simulink library "legs"  (R2020b)
settings: Solver=VariableStepAuto  StartTime=0.0  StopTime=10.0  RelTol=1e-3
values from neighbouring files (symbols this model uses):
  N = size(waypoints, 1)    [interpolate_leg_waypoints.m]
undefined symbols (not defined in the file or in its folder): beta, X, Y, Z
libraries: sm_lib x42, $bdroot x21, nesl_utility x9
(part 1 of 2)
settings Model: Creator=zach  LastModifiedBy=zach

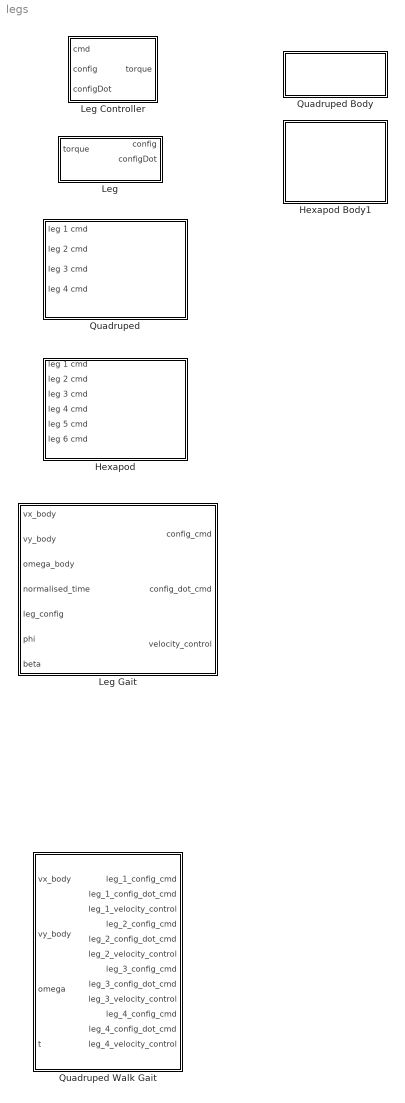
== system legs ==
  Hexapod : Subsystem  AncestorBlock=legs/Quadruped
  Hexapod Body1 : Subsystem  AncestorBlock=legs/Quadruped Body  mask{radius=0.5, height=0.1, leg_radius=0.02, mass=0}
      mask prompts: leg_radius "Leg Radius"
  Leg : Subsystem  mask{length_1=0.1, length_2=0.3, length_3=0.3, radius=0.04, mass_1=0.1, mass_2=0.3, mass_3=0.3}
      mask prompts: length_1 "Length 1"; length_2 "Length 2"; length_3 "Length 3"; mass_1 "Mass 1"; mass_2 "Mass 2"; mass_3 "Mass 3"
  Leg Controller : Subsystem  mask{kp=[10; 10; 10], ki=[1; 1; 1], kd=[0.1; 0.1; 0.1]}
  Leg Gait : Subsystem  mask{distance=0.3, rotation_z=0, contact_start_config=[0; pi/4; pi/4]}
      mask prompts: rotation_z "Rotation Z"; contact_start_config "Leg config at start of contact phase"
  Quadruped : Subsystem
  Quadruped Body : Subsystem  mask{length=0.4, width=0.3, height=0.1, leg_radius=0.04, mass=0}
      mask prompts: leg_radius "Leg Radius"
  Quadruped Walk Gait : Subsystem  mask{T=1}
      mask prompts: T "Period"

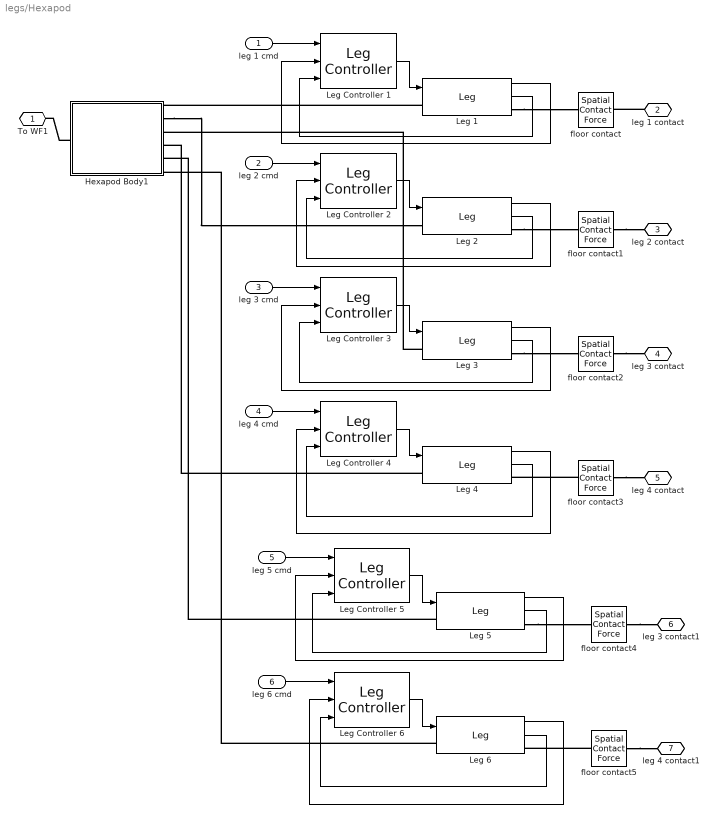
== system legs/Hexapod ==
  leg 1 cmd : Inport
  leg 2 cmd : Inport  Port=2
  leg 3 cmd : Inport  Port=3
  leg 4 cmd : Inport  Port=4
  leg 5 cmd : Inport  Port=5
  leg 6 cmd : Inport  Port=6
  Hexapod Body1 : Subsystem  AncestorBlock=legs/Quadruped Body  mask{radius=0.5, height=0.1, leg_radius=0.02, mass=0}
      mask prompts: leg_radius "Leg Radius"
  Leg {1..6} (6 alike) : $bdroot/Leg  length_1=0.1  length_2=0.3  length_3=0.3  radius=0.02  mass_1=0.1  mass_2=0.3  mass_3=0.3
  Leg Controller {1..6} (6 alike) : $bdroot/Leg Controller  kp=[20; 20; 20]  ki=[5; 5; 5]  kd=[1; 1; 1]
  floor contact{,1..5} (6 alike) : sm_lib/Forces and Torques/Spatial Contact Force  CoefficientOfDynamicFriction=0.3  CoefficientOfStaticFriction=1  NormalDamping=1e3  NormalDampingUnits=N/(m/s)  NormalStiffness=1e6  NormalStiffnessUnits=N/m  FrictionalCriticalVelocity=1e-3  FrictionalCriticalVelocityUnits=m/s  ZeroCrossDetectContactStartAndEnd=off  SenseFrictionalForceMagnitude=off  SenseNormalForceMagnitude=off  SenseSeparationDistance=off  NormalTransitionRegionWidth=1e-4  NormalTransitionRegionWidthUnits=m  FrictionType=SmoothStickSlip
  To WF1 : PMIOPort  Side=Left
  leg 1 contact : PMIOPort  Port=2  Side=Right
  leg 2 contact : PMIOPort  Port=3  Side=Right
  leg 3 contact : PMIOPort  Port=4  Side=Right
  leg 4 contact : PMIOPort  Port=5  Side=Right
  leg 3 contact1 : PMIOPort  Port=6  Side=Right
  leg 4 contact1 : PMIOPort  Port=7  Side=Right
  wires:
  Leg 2/2 -> Leg Controller 2/3
  Leg 2/1 -> Leg Controller 2/2
  Leg 1/1 -> Leg Controller 1/2
  leg 2 cmd/1 -> Leg Controller 2/1
  Leg 3/2 -> Leg Controller 3/3
  leg 4 cmd/1 -> Leg Controller 4/1
  leg 1 cmd/1 -> Leg Controller 1/1
  leg 3 cmd/1 -> Leg Controller 3/1
  Leg 4/1 -> Leg Controller 4/2
  Leg Controller 4/1 -> Leg 4/1
  Leg 4/2 -> Leg Controller 4/3
  Leg 3/1 -> Leg Controller 3/2
  Leg Controller 1/1 -> Leg 1/1
  Leg 1/2 -> Leg Controller 1/3
  Leg Controller 3/1 -> Leg 3/1
  Leg Controller 2/1 -> Leg 2/1
  Leg Controller 5/1 -> Leg 5/1
  Leg 6/1 -> Leg Controller 6/2
  leg 5 cmd/1 -> Leg Controller 5/1
  Leg Controller 6/1 -> Leg 6/1
  Leg 6/2 -> Leg Controller 6/3
  Leg 5/2 -> Leg Controller 5/3
  leg 6 cmd/1 -> Leg Controller 6/1
  Leg 5/1 -> Leg Controller 5/2
  connections:
  floor contact1/RConn1 -- leg 2 contact/RConn1
  floor contact3/RConn1 -- leg 4 contact/RConn1
  floor contact2/RConn1 -- leg 3 contact/RConn1
  leg 1 contact/RConn1 -- floor contact/RConn1
  Leg 1/RConn1 -- floor contact/LConn1
  Leg 3/LConn1 -- Hexapod Body1/RConn3
  Hexapod Body1/RConn2 -- Leg 2/LConn1
  Leg 1/LConn1 -- Hexapod Body1/RConn1
  Leg 4/LConn1 -- Hexapod Body1/RConn4
  Leg 2/RConn1 -- floor contact1/LConn1
  floor contact3/LConn1 -- Leg 4/RConn1
  Leg 3/RConn1 -- floor contact2/LConn1
  Hexapod Body1/LConn1 -- To WF1/RConn1
  floor contact4/RConn1 -- leg 3 contact1/RConn1
  floor contact5/RConn1 -- leg 4 contact1/RConn1
  Leg 6/LConn1 -- Hexapod Body1/RConn6
  Leg 5/RConn1 -- floor contact4/LConn1
  floor contact5/LConn1 -- Leg 6/RConn1
  Leg 5/LConn1 -- Hexapod Body1/RConn5

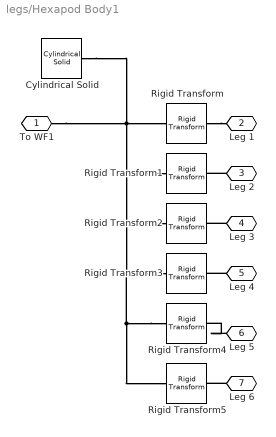
== system legs/Hexapod Body1 ==
  Cylindrical Solid : sm_lib/Body Elements/Cylindrical Solid  GraphicAmbientColor=[0.15 0.15 0.15 1.0]  BasedOnType=Density  CenterOfMass=[0 0 0]  CenterOfMassUnits=m  GraphicDiffuseColor=[0.5 0.5 0.5]  CylinderLength=height  CylinderLengthUnits=m  CylinderRadius=radius  CylinderRadiusUnits=m  Density=1000  DensityUnits=kg/m^3  DoExposeReferenceFrame=on  GraphicEmissiveColor=[0.0 0.0 0.0 1.0]  ExportEntireGeometry=off  SerializedFrames=<Frames/>  MarkerShape=Sphere  MarkerSize=10  GraphicType=FromGeometry  InertiaType=CalculateFromGeometry  Mass=1  MassUnits=kg  MomentsOfInertia=[1 1 1]  MomentsOfInertiaUnits=kg*m^2  GraphicOpacity=1.0  ProductsOfInertia=[0 0 0]  ProductsOfInertiaUnits=kg*m^2  GraphicShininess=75  GraphicSpecularColor=[0.5 0.5 0.5 1.0]  GraphicVisPropType=SimpleVisualProperties
  Rigid Transform : sm_lib/Frames and Transforms/Rigid Transform  TranslationMethod=Cylindrical  TranslationStandardOffset=0  TranslationLengthUnit=m  TranslationStandardAxis=+Z  TranslationCartesianOffset=[radius*cos(1/3*pi) radius*sin(1/3*pi) 0]  TranslationROffset=radius  TranslationROffsetUnits=m  TranslationZOffset=0  TranslationZOffsetUnits=m  TranslationThetaOffset=60  TranslationThetaOffsetUnits=deg  RotationMethod=StandardAxis  RotationAngleUnits=deg  RotationStandardAxis=+Z  RotationAngle=60  RotationArbitraryAxis=[0 0 1]  FollAlignAxisA=+X  BaseAlignAxisA=+Y  FollAlignAxisB=+Y  BaseAlignAxisB=+Z  RotationSequenceAxes=FollowerAxes  RotationSequence=XYX  RotationSequenceAngles=[0 0 0]  RotationSequenceAnglesUnits=deg  RotationMatrix=[1 0 0; 0 1 0; 0 0 1]
  Rigid Transform1 : sm_lib/Frames and Transforms/Rigid Transform  TranslationMethod=Cartesian  TranslationStandardOffset=0  TranslationLengthUnit=m  TranslationStandardAxis=+Z  TranslationCartesianOffset=[radius*cos(2/3*pi) radius*sin(2/3*pi) 0]  TranslationROffset=0  TranslationROffsetUnits=m  TranslationZOffset=0  TranslationZOffsetUnits=m  TranslationThetaOffset=0  TranslationThetaOffsetUnits=deg  RotationMethod=StandardAxis  RotationAngleUnits=rad  RotationStandardAxis=+Z  RotationAngle=2/3*pi  RotationArbitraryAxis=[0 0 1]  FollAlignAxisA=+X  BaseAlignAxisA=+Y  FollAlignAxisB=+Y  BaseAlignAxisB=+Z  RotationSequenceAxes=FollowerAxes  RotationSequence=XYX  RotationSequenceAngles=[0 0 0]  RotationSequenceAnglesUnits=deg  RotationMatrix=[1 0 0; 0 1 0; 0 0 1]
  Rigid Transform2 : sm_lib/Frames and Transforms/Rigid Transform  TranslationMethod=Cartesian  TranslationStandardOffset=0  TranslationLengthUnit=m  TranslationStandardAxis=+Z  TranslationCartesianOffset=[radius*cos(pi) radius*sin(pi) 0]  TranslationROffset=0  TranslationROffsetUnits=m  TranslationZOffset=0  TranslationZOffsetUnits=m  TranslationThetaOffset=0  TranslationThetaOffsetUnits=deg  RotationMethod=StandardAxis  RotationAngleUnits=rad  RotationStandardAxis=+Z  RotationAngle=pi  RotationArbitraryAxis=[0 0 1]  FollAlignAxisA=+X  BaseAlignAxisA=+Y  FollAlignAxisB=+Y  BaseAlignAxisB=+Z  RotationSequenceAxes=FollowerAxes  RotationSequence=XYX  RotationSequenceAngles=[0 0 0]  RotationSequenceAnglesUnits=deg  RotationMatrix=[1 0 0; 0 1 0; 0 0 1]
  Rigid Transform3 : sm_lib/Frames and Transforms/Rigid Transform  TranslationMethod=Cartesian  TranslationStandardOffset=0  TranslationLengthUnit=m  TranslationStandardAxis=+Z  TranslationCartesianOffset=[radius*cos(4/3*pi) radius*sin(4/3*pi) 0]  TranslationROffset=0  TranslationROffsetUnits=m  TranslationZOffset=0  TranslationZOffsetUnits=m  TranslationThetaOffset=0  TranslationThetaOffsetUnits=deg  RotationMethod=StandardAxis  RotationAngleUnits=rad  RotationStandardAxis=+Z  RotationAngle=4/3*pi  RotationArbitraryAxis=[0 0 1]  FollAlignAxisA=+X  BaseAlignAxisA=+Y  FollAlignAxisB=+Y  BaseAlignAxisB=+Z  RotationSequenceAxes=FollowerAxes  RotationSequence=XYX  RotationSequenceAngles=[0 0 0]  RotationSequenceAnglesUnits=deg  RotationMatrix=[1 0 0; 0 1 0; 0 0 1]
  Rigid Transform4 : sm_lib/Frames and Transforms/Rigid Transform  TranslationMethod=Cartesian  TranslationStandardOffset=0  TranslationLengthUnit=m  TranslationStandardAxis=+Z  TranslationCartesianOffset=[radius*cos(5/3*pi) radius*sin(5/3*pi) 0]  TranslationROffset=0  TranslationROffsetUnits=m  TranslationZOffset=0  TranslationZOffsetUnits=m  TranslationThetaOffset=0  TranslationThetaOffsetUnits=deg  RotationMethod=StandardAxis  RotationAngleUnits=rad  RotationStandardAxis=+Z  RotationAngle=5/3*pi  RotationArbitraryAxis=[0 0 1]  FollAlignAxisA=+X  BaseAlignAxisA=+Y  FollAlignAxisB=+Y  BaseAlignAxisB=+Z  RotationSequenceAxes=FollowerAxes  RotationSequence=XYX  RotationSequenceAngles=[0 0 0]  RotationSequenceAnglesUnits=deg  RotationMatrix=[1 0 0; 0 1 0; 0 0 1]
  Rigid Transform5 : sm_lib/Frames and Transforms/Rigid Transform  TranslationMethod=Cartesian  TranslationStandardOffset=0  TranslationLengthUnit=m  TranslationStandardAxis=+Z  TranslationCartesianOffset=[radius*cos(2*pi) radius*sin(2*pi) 0]  TranslationROffset=0  TranslationROffsetUnits=m  TranslationZOffset=0  TranslationZOffsetUnits=m  TranslationThetaOffset=0  TranslationThetaOffsetUnits=deg  RotationMethod=StandardAxis  RotationAngleUnits=rad  RotationStandardAxis=+Z  RotationAngle=2*pi  RotationArbitraryAxis=[0 0 1]  FollAlignAxisA=+X  BaseAlignAxisA=+Y  FollAlignAxisB=+Y  BaseAlignAxisB=+Z  RotationSequenceAxes=FollowerAxes  RotationSequence=XYX  RotationSequenceAngles=[0 0 0]  RotationSequenceAnglesUnits=deg  RotationMatrix=[1 0 0; 0 1 0; 0 0 1]
  To WF1 : PMIOPort  Side=Left
  Leg 1 : PMIOPort  Port=2  Side=Right
  Leg 2 : PMIOPort  Port=3  Side=Right
  Leg 3 : PMIOPort  Port=4  Side=Right
  Leg 4 : PMIOPort  Port=5  Side=Right
  Leg 5 : PMIOPort  Port=6  Side=Right
  Leg 6 : PMIOPort  Port=7  Side=Right
  connections:
  Rigid Transform/RConn1 -- Leg 1/RConn1
  Rigid Transform4/LConn1 -- Rigid Transform5/LConn1 -- To WF1/RConn1 -- Cylindrical Solid/RConn1 -- Rigid Transform/LConn1 -- Rigid Transform1/LConn1 -- Rigid Transform2/LConn1 -- Rigid Transform3/LConn1
  Leg 2/RConn1 -- Rigid Transform1/RConn1
  Leg 4/RConn1 -- Rigid Transform3/RConn1
  Leg 3/RConn1 -- Rigid Transform2/RConn1
  Leg 5/RConn1 -- Rigid Transform4/RConn1
  Leg 6/RConn1 -- Rigid Transform5/RConn1

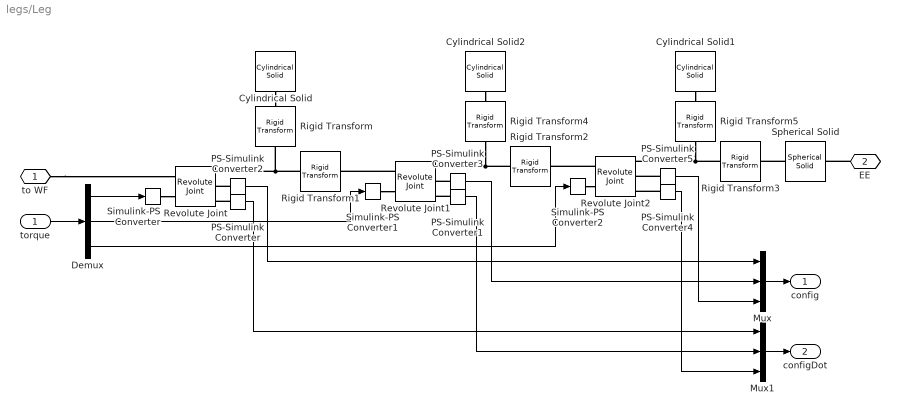
== system legs/Leg ==
  torque : Inport  PortDimensions=3
  Cylindrical Solid : sm_lib/Body Elements/Cylindrical Solid  GraphicAmbientColor=[0.15 0.15 0.15 1.0]  BasedOnType=Mass  CenterOfMass=[0 0 0]  CenterOfMassUnits=m  GraphicDiffuseColor=[0.2 0.2 0.2]  CylinderLength=length_1  CylinderLengthUnits=m  CylinderRadius=radius  CylinderRadiusUnits=m  Density=1000  DensityUnits=kg/m^3  DoExposeReferenceFrame=on  GraphicEmissiveColor=[0.0 0.0 0.0 1.0]  ExportEntireGeometry=off  SerializedFrames=<Frames/>  MarkerShape=Sphere  MarkerSize=10  GraphicType=FromGeometry  InertiaType=CalculateFromGeometry  Mass=mass_1  MassUnits=kg  MomentsOfInertia=[1 1 1]  MomentsOfInertiaUnits=kg*m^2  GraphicOpacity=1.0  ProductsOfInertia=[0 0 0]  ProductsOfInertiaUnits=kg*m^2  GraphicShininess=75  GraphicSpecularColor=[0.5 0.5 0.5 1.0]  GraphicVisPropType=SimpleVisualProperties
  Cylindrical Solid1 : sm_lib/Body Elements/Cylindrical Solid  GraphicAmbientColor=[0.15 0.15 0.15 1.0]  BasedOnType=Mass  CenterOfMass=[0 0 0]  CenterOfMassUnits=m  GraphicDiffuseColor=[0.2 0.2 0.2]  CylinderLength=length_3  CylinderLengthUnits=m  CylinderRadius=radius  CylinderRadiusUnits=m  Density=1000  DensityUnits=kg/m^3  DoExposeReferenceFrame=on  GraphicEmissiveColor=[0.0 0.0 0.0 1.0]  ExportEntireGeometry=off  SerializedFrames=<Frames/>  MarkerShape=Sphere  MarkerSize=10  GraphicType=FromGeometry  InertiaType=CalculateFromGeometry  Mass=mass_3  MassUnits=kg  MomentsOfInertia=[1 1 1]  MomentsOfInertiaUnits=kg*m^2  GraphicOpacity=1.0  ProductsOfInertia=[0 0 0]  ProductsOfInertiaUnits=kg*m^2  GraphicShininess=75  GraphicSpecularColor=[0.5 0.5 0.5 1.0]  GraphicVisPropType=SimpleVisualProperties
  Cylindrical Solid2 : sm_lib/Body Elements/Cylindrical Solid  GraphicAmbientColor=[0.15 0.15 0.15 1.0]  BasedOnType=Mass  CenterOfMass=[0 0 0]  CenterOfMassUnits=m  GraphicDiffuseColor=[0.2 0.2 0.2]  CylinderLength=length_2  CylinderLengthUnits=m  CylinderRadius=radius  CylinderRadiusUnits=m  Density=1000  DensityUnits=kg/m^3  DoExposeReferenceFrame=on  GraphicEmissiveColor=[0.0 0.0 0.0 1.0]  ExportEntireGeometry=off  SerializedFrames=<Frames/>  MarkerShape=Sphere  MarkerSize=10  GraphicType=FromGeometry  InertiaType=CalculateFromGeometry  Mass=mass_2  MassUnits=kg  MomentsOfInertia=[1 1 1]  MomentsOfInertiaUnits=kg*m^2  GraphicOpacity=1.0  ProductsOfInertia=[0 0 0]  ProductsOfInertiaUnits=kg*m^2  GraphicShininess=75  GraphicSpecularColor=[0.5 0.5 0.5 1.0]  GraphicVisPropType=SimpleVisualProperties
  Demux : Demux  Outputs=3
  Mux : Mux  Inputs=3
  Mux1 : Mux  Inputs=3
  PS-Simulink Converter{,1..5} (6 alike) : nesl_utility/PS-Simulink Converter  PhysicalDomain=network_engine_domain  SubClassName=ps_output  LeftPortType=input  RightPortType=output  PseudoPeriodic=off  Frequencies=[]  Unit=inherit  AffineConversion=off
  Revolute Joint : sm_lib/Joints/Revolute Joint  JointMode=Normal  SenseConstraintForce=off  SenseConstraintForceX=off  SenseConstraintForceY=off  SenseConstraintForceZ=off  SenseConstraintTorque=off  SenseConstraintTorqueX=off  SenseConstraintTorqueY=off  SenseConstraintTorqueZ=off  SenseTotalForce=off  SenseTotalForceX=off  SenseTotalForceY=off  SenseTotalForceZ=off  SenseTotalTorque=off  SenseTotalTorqueX=off  SenseTotalTorqueY=off  SenseTotalTorqueZ=off  CompositeWrenchDir=FollowerOnBase  CompositeWrenchFrame=BaseFrame  EquilibriumPosition=0  EquilibriumPositionUnits=deg  SpringStiffness=0  SpringStiffnessUnits=N*m/deg  DampingCoefficient=0  DampingCoefficientUnits=N*m/(deg/s)  TorqueActuationMode=InputTorque  MotionActuationMode=ComputedMotion  SensePosition=on  SenseVelocity=on  SenseAcceleration=off  SenseTorqueForce=off  SenseLowerLimitTorqueForce=off  SenseUpperLimitTorqueForce=off  LowerLimitSpecify=off  LowerLimitBound=-90  LowerLimitBoundUnits=deg  LowerLimitStiffness=1e4  LowerLimitStiffnessUnits=N*m/deg  LowerLimitDamping=10  LowerLimitDampingUnits=N*m/(deg/s)  LowerLimitTransitionRegionWidth=0.1  LowerLimitTransitionRegionWidthUnits=deg  UpperLimitSpecify=off  UpperLimitBound=90  UpperLimitBoundUnits=deg  UpperLimitStiffness=1e4  UpperLimitStiffnessUnits=N*m/deg  UpperLimitDamping=10  UpperLimitDampingUnits=N*m/(deg/s)  UpperLimitTransitionRegionWidth=0.1  UpperLimitTransitionRegionWidthUnits=deg  PositionTargetSpecify=on  PositionTargetPriority=High  PositionTargetValue=0  PositionTargetValueUnits=rad  VelocityTargetSpecify=on  VelocityTargetPriority=High  VelocityTargetValue=0  VelocityTargetValueUnits=deg/s
  Revolute Joint1 : sm_lib/Joints/Revolute Joint  JointMode=Normal  SenseConstraintForce=off  SenseConstraintForceX=off  SenseConstraintForceY=off  SenseConstraintForceZ=off  SenseConstraintTorque=off  SenseConstraintTorqueX=off  SenseConstraintTorqueY=off  SenseConstraintTorqueZ=off  SenseTotalForce=off  SenseTotalForceX=off  SenseTotalForceY=off  SenseTotalForceZ=off  SenseTotalTorque=off  SenseTotalTorqueX=off  SenseTotalTorqueY=off  SenseTotalTorqueZ=off  CompositeWrenchDir=FollowerOnBase  CompositeWrenchFrame=BaseFrame  EquilibriumPosition=0  EquilibriumPositionUnits=deg  SpringStiffness=0  SpringStiffnessUnits=N*m/deg  DampingCoefficient=0  DampingCoefficientUnits=N*m/(deg/s)  TorqueActuationMode=InputTorque  MotionActuationMode=ComputedMotion  SensePosition=on  SenseVelocity=on  SenseAcceleration=off  SenseTorqueForce=off  SenseLowerLimitTorqueForce=off  SenseUpperLimitTorqueForce=off  LowerLimitSpecify=off  LowerLimitBound=-90  LowerLimitBoundUnits=deg  LowerLimitStiffness=1e4  LowerLimitStiffnessUnits=N*m/deg  LowerLimitDamping=10  LowerLimitDampingUnits=N*m/(deg/s)  LowerLimitTransitionRegionWidth=0.1  LowerLimitTransitionRegionWidthUnits=deg  UpperLimitSpecify=off  UpperLimitBound=90  UpperLimitBoundUnits=deg  UpperLimitStiffness=1e4  UpperLimitStiffnessUnits=N*m/deg  UpperLimitDamping=10  UpperLimitDampingUnits=N*m/(deg/s)  UpperLimitTransitionRegionWidth=0.1  UpperLimitTransitionRegionWidthUnits=deg  PositionTargetSpecify=on  PositionTargetPriority=High  PositionTargetValue=0  PositionTargetValueUnits=rad  VelocityTargetSpecify=on  VelocityTargetPriority=High  VelocityTargetValue=0  VelocityTargetValueUnits=deg/s
  Revolute Joint2 : sm_lib/Joints/Revolute Joint  JointMode=Normal  SenseConstraintForce=off  SenseConstraintForceX=off  SenseConstraintForceY=off  SenseConstraintForceZ=off  SenseConstraintTorque=off  SenseConstraintTorqueX=off  SenseConstraintTorqueY=off  SenseConstraintTorqueZ=off  SenseTotalForce=off  SenseTotalForceX=off  SenseTotalForceY=off  SenseTotalForceZ=off  SenseTotalTorque=off  SenseTotalTorqueX=off  SenseTotalTorqueY=off  SenseTotalTorqueZ=off  CompositeWrenchDir=FollowerOnBase  CompositeWrenchFrame=BaseFrame  EquilibriumPosition=0  EquilibriumPositionUnits=deg  SpringStiffness=0  SpringStiffnessUnits=N*m/deg  DampingCoefficient=0  DampingCoefficientUnits=N*m/(deg/s)  TorqueActuationMode=InputTorque  MotionActuationMode=ComputedMotion  SensePosition=on  SenseVelocity=on  SenseAcceleration=off  SenseTorqueForce=off  SenseLowerLimitTorqueForce=off  SenseUpperLimitTorqueForce=off  LowerLimitSpecify=off  LowerLimitBound=-90  LowerLimitBoundUnits=deg  LowerLimitStiffness=1e4  LowerLimitStiffnessUnits=N*m/deg  LowerLimitDamping=10  LowerLimitDampingUnits=N*m/(deg/s)  LowerLimitTransitionRegionWidth=0.1  LowerLimitTransitionRegionWidthUnits=deg  UpperLimitSpecify=off  UpperLimitBound=90  UpperLimitBoundUnits=deg  UpperLimitStiffness=1e4  UpperLimitStiffnessUnits=N*m/deg  UpperLimitDamping=10  UpperLimitDampingUnits=N*m/(deg/s)  UpperLimitTransitionRegionWidth=0.1  UpperLimitTransitionRegionWidthUnits=deg  PositionTargetSpecify=on  PositionTargetPriority=High  PositionTargetValue=0  PositionTargetValueUnits=rad  VelocityTargetSpecify=on  VelocityTargetPriority=High  VelocityTargetValue=0  VelocityTargetValueUnits=deg/s
  Rigid Transform : sm_lib/Frames and Transforms/Rigid Transform  TranslationMethod=StandardAxis  TranslationStandardOffset=length_1/2  TranslationLengthUnit=m  TranslationStandardAxis=+Z  TranslationCartesianOffset=[0 0 0]  TranslationROffset=0  TranslationROffsetUnits=m  TranslationZOffset=0  TranslationZOffsetUnits=m  TranslationThetaOffset=0  TranslationThetaOffsetUnits=deg  RotationMethod=StandardAxis  RotationAngleUnits=deg  RotationStandardAxis=+Y  RotationAngle=90  RotationArbitraryAxis=[0 0 1]  FollAlignAxisA=+X  BaseAlignAxisA=+Y  FollAlignAxisB=+Y  BaseAlignAxisB=+Z  RotationSequenceAxes=FollowerAxes  RotationSequence=XYX  RotationSequenceAngles=[0 0 0]  RotationSequenceAnglesUnits=deg  RotationMatrix=[1 0 0; 0 1 0; 0 0 1]
  Rigid Transform1 : sm_lib/Frames and Transforms/Rigid Transform  TranslationMethod=StandardAxis  TranslationStandardOffset=length_1  TranslationLengthUnit=m  TranslationStandardAxis=+X  TranslationCartesianOffset=[0.1 0 0]  TranslationROffset=0  TranslationROffsetUnits=m  TranslationZOffset=0  TranslationZOffsetUnits=m  TranslationThetaOffset=0  TranslationThetaOffsetUnits=deg  RotationMethod=StandardAxis  RotationAngleUnits=deg  RotationStandardAxis=-X  RotationAngle=90  RotationArbitraryAxis=[0 0 1]  FollAlignAxisA=+X  BaseAlignAxisA=+Y  FollAlignAxisB=+Y  BaseAlignAxisB=+Z  RotationSequenceAxes=FollowerAxes  RotationSequence=XYX  RotationSequenceAngles=[0 0 0]  RotationSequenceAnglesUnits=deg  RotationMatrix=[1 0 0; 0 1 0; 0 0 1]
  Rigid Transform2 : sm_lib/Frames and Transforms/Rigid Transform  TranslationMethod=StandardAxis  TranslationStandardOffset=length_2  TranslationLengthUnit=m  TranslationStandardAxis=+X  TranslationCartesianOffset=[0 0 0]  TranslationROffset=0  TranslationROffsetUnits=m  TranslationZOffset=0  TranslationZOffsetUnits=m  TranslationThetaOffset=0  TranslationThetaOffsetUnits=deg  RotationMethod=None  RotationAngleUnits=deg  RotationStandardAxis=+X  RotationAngle=90  RotationArbitraryAxis=[0 0 1]  FollAlignAxisA=+X  BaseAlignAxisA=+Y  FollAlignAxisB=+Y  BaseAlignAxisB=+Z  RotationSequenceAxes=FollowerAxes  RotationSequence=XYX  RotationSequenceAngles=[0 0 0]  RotationSequenceAnglesUnits=deg  RotationMatrix=[1 0 0; 0 1 0; 0 0 1]
  Rigid Transform3 : sm_lib/Frames and Transforms/Rigid Transform  TranslationMethod=StandardAxis  TranslationStandardOffset=length_3  TranslationLengthUnit=m  TranslationStandardAxis=+X  TranslationCartesianOffset=[0 0 0]  TranslationROffset=0  TranslationROffsetUnits=m  TranslationZOffset=0  TranslationZOffsetUnits=m  TranslationThetaOffset=0  TranslationThetaOffsetUnits=deg  RotationMethod=None  RotationAngleUnits=deg  RotationStandardAxis=+X  RotationAngle=90  RotationArbitraryAxis=[0 0 1]  FollAlignAxisA=+X  BaseAlignAxisA=+Y  FollAlignAxisB=+Y  BaseAlignAxisB=+Z  RotationSequenceAxes=FollowerAxes  RotationSequence=XYX  RotationSequenceAngles=[0 0 0]  RotationSequenceAnglesUnits=deg  RotationMatrix=[1 0 0; 0 1 0; 0 0 1]
  Rigid Transform4 : sm_lib/Frames and Transforms/Rigid Transform  TranslationMethod=StandardAxis  TranslationStandardOffset=length_2/2  TranslationLengthUnit=m  TranslationStandardAxis=+Z  TranslationCartesianOffset=[0 0 0]  TranslationROffset=0  TranslationROffsetUnits=m  TranslationZOffset=0  TranslationZOffsetUnits=m  TranslationThetaOffset=0  TranslationThetaOffsetUnits=deg  RotationMethod=StandardAxis  RotationAngleUnits=deg  RotationStandardAxis=+Y  RotationAngle=90  RotationArbitraryAxis=[0 0 1]  FollAlignAxisA=+X  BaseAlignAxisA=+Y  FollAlignAxisB=+Y  BaseAlignAxisB=+Z  RotationSequenceAxes=FollowerAxes  RotationSequence=XYX  RotationSequenceAngles=[0 0 0]  RotationSequenceAnglesUnits=deg  RotationMatrix=[1 0 0; 0 1 0; 0 0 1]
  Rigid Transform5 : sm_lib/Frames and Transforms/Rigid Transform  TranslationMethod=StandardAxis  TranslationStandardOffset=length_3/2  TranslationLengthUnit=m  TranslationStandardAxis=+Z  TranslationCartesianOffset=[0 0 0]  TranslationROffset=0  TranslationROffsetUnits=m  TranslationZOffset=0  TranslationZOffsetUnits=m  TranslationThetaOffset=0  TranslationThetaOffsetUnits=deg  RotationMethod=StandardAxis  RotationAngleUnits=deg  RotationStandardAxis=+Y  RotationAngle=90  RotationArbitraryAxis=[0 0 1]  FollAlignAxisA=+X  BaseAlignAxisA=+Y  FollAlignAxisB=+Y  BaseAlignAxisB=+Z  RotationSequenceAxes=FollowerAxes  RotationSequence=XYX  RotationSequenceAngles=[0 0 0]  RotationSequenceAnglesUnits=deg  RotationMatrix=[1 0 0; 0 1 0; 0 0 1]
  Simulink-PS Converter : nesl_utility/Simulink-PS Converter  PhysicalDomain=network_engine_domain  SubClassName=ps_input  LeftPortType=input  RightPortType=output  PseudoPeriodic=off  Frequencies=[]  NoiseDistribution=none  NoiseParameters=[]  Unit=1  AffineConversion=off  FilteringAndDerivatives=filter  SimscapeFilterOrder=2  InputFilterTimeConstant=0.001  UdotUserProvided=0
  Simulink-PS Converter1 : nesl_utility/Simulink-PS Converter  PhysicalDomain=network_engine_domain  SubClassName=ps_input  LeftPortType=input  RightPortType=output  PseudoPeriodic=off  Frequencies=[]  NoiseDistribution=none  NoiseParameters=[]  Unit=1  AffineConversion=off  FilteringAndDerivatives=filter  SimscapeFilterOrder=2  InputFilterTimeConstant=0.001  UdotUserProvided=0
  Simulink-PS Converter2 : nesl_utility/Simulink-PS Converter  PhysicalDomain=network_engine_domain  SubClassName=ps_input  LeftPortType=input  RightPortType=output  PseudoPeriodic=off  Frequencies=[]  NoiseDistribution=none  NoiseParameters=[]  Unit=1  AffineConversion=off  FilteringAndDerivatives=filter  SimscapeFilterOrder=2  InputFilterTimeConstant=0.001  UdotUserProvided=0
  Spherical Solid : sm_lib/Body Elements/Spherical Solid  GraphicAmbientColor=[0.15 0.15 0.15 1.0]  BasedOnType=Density  CenterOfMass=[0 0 0]  CenterOfMassUnits=m  GraphicDiffuseColor=[0.5 0.5 0.5]  Density=1000  DensityUnits=kg/m^3  DoExposeReferenceFrame=on  GraphicEmissiveColor=[0.0 0.0 0.0 1.0]  ExportEntireGeometry=on  SerializedExposedGeometries=<ExposedGeometries><ExposedGeometry><RawGeometryId>entire</RawGeometryId><ExposedGeometryId>G</ExposedGeometryId></ExposedGeometry></ExposedGeometries>  SerializedFrames=<Frames/>  MarkerShape=Sphere  MarkerSize=10  GraphicType=FromGeometry  InertiaType=CalculateFromGeometry  Mass=1  MassUnits=kg  MomentsOfInertia=[1 1 1]  MomentsOfInertiaUnits=kg*m^2  GraphicOpacity=1.0  ProductsOfInertia=[0 0 0]  ProductsOfInertiaUnits=kg*m^2  GraphicShininess=75  GraphicSpecularColor=[0.5 0.5 0.5 1.0]  SphereRadius=radius  SphereRadiusUnits=m  GraphicVisPropType=SimpleVisualProperties
  to WF : PMIOPort  Side=Left
  EE : PMIOPort  Port=2  Side=Right
  config : Outport
  configDot : Outport  Port=2
  wires:
  torque/1 -> Demux/1
  Mux1/1 -> configDot/1
  Mux/1 -> config/1
  Demux/1 -> Simulink-PS Converter/1
  PS-Simulink Converter2/1 -> Mux/1
  PS-Simulink Converter/1 -> Mux1/1
  Demux/2 -> Simulink-PS Converter1/1
  PS-Simulink Converter1/1 -> Mux1/2
  PS-Simulink Converter3/1 -> Mux/2
  Demux/3 -> Simulink-PS Converter2/1
  PS-Simulink Converter4/1 -> Mux1/3
  PS-Simulink Converter5/1 -> Mux/3
  connections:
  Rigid Transform1/LConn1 -- Rigid Transform/RConn1 -- Revolute Joint/RConn1
  Cylindrical Solid2/RConn1 -- Rigid Transform4/LConn1
  Simulink-PS Converter/RConn1 -- Revolute Joint/LConn2
  to WF/RConn1 -- Revolute Joint/LConn1
  PS-Simulink Converter/LConn1 -- Revolute Joint/RConn3
  PS-Simulink Converter2/LConn1 -- Revolute Joint/RConn2
  PS-Simulink Converter3/LConn1 -- Revolute Joint1/RConn2
  Simulink-PS Converter1/RConn1 -- Revolute Joint1/LConn2
  PS-Simulink Converter1/LConn1 -- Revolute Joint1/RConn3
  Revolute Joint1/LConn1 -- Rigid Transform1/RConn1
  Rigid Transform3/LConn1 -- Rigid Transform5/RConn1 -- Revolute Joint2/RConn1
  PS-Simulink Converter4/LConn1 -- Revolute Joint2/RConn3
  Simulink-PS Converter2/RConn1 -- Revolute Joint2/LConn2
  PS-Simulink Converter5/LConn1 -- Revolute Joint2/RConn2
  Revolute Joint2/LConn1 -- Rigid Transform2/RConn1
  Cylindrical Solid/RConn1 -- Rigid Transform/LConn1
  Rigid Transform4/RConn1 -- Revolute Joint1/RConn1 -- Rigid Transform2/LConn1
  Cylindrical Solid1/RConn1 -- Rigid Transform5/LConn1
  Spherical Solid/RConn1 -- Rigid Transform3/RConn1
  EE/RConn1 -- Spherical Solid/LConn1

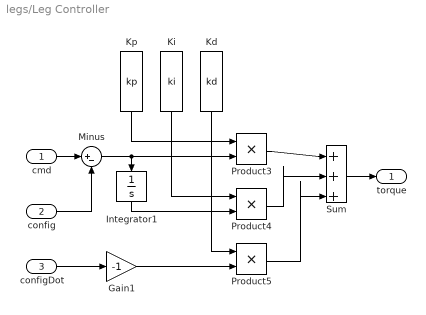
== system legs/Leg Controller ==
  cmd : Inport
  config : Inport  Port=2
  configDot : Inport  Port=3
  Gain1 : Gain  Gain=-1
  Integrator1 : Integrator
  Kd : Constant  Value=kd
  Ki : Constant  Value=ki
  Kp : Constant  Value=kp
  Minus : Sum  Inputs=|+-
  Product3 : Product
  Product4 : Product
  Product5 : Product
  Sum : Sum  Inputs=+++|
  torque : Outport
  wires:
  cmd/1 -> Minus/1
  config/1 -> Minus/2
  Minus/1 -> Product3/2, Integrator1/1
  Integrator1/1 -> Product4/2
  configDot/1 -> Gain1/1
  Gain1/1 -> Product5/2
  Kd/1 -> Product5/1
  Ki/1 -> Product4/1
  Kp/1 -> Product3/1
  Sum/1 -> torque/1
  Product3/1 -> Sum/1
  Product4/1 -> Sum/2
  Product5/1 -> Sum/3

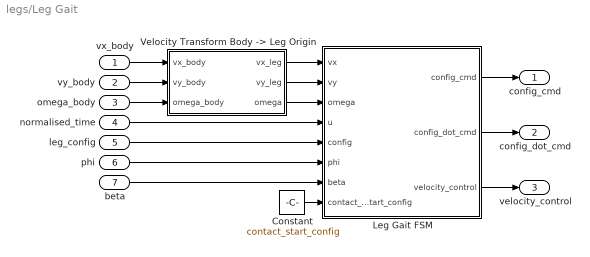
== system legs/Leg Gait ==
  vx_body : Inport
  vy_body : Inport  Port=2
  omega_body : Inport  Port=3
  normalised_time : Inport  Port=4
  leg_config : Inport  Port=5
  phi : Inport  Port=6
  beta : Inport  Port=7
  Constant : Constant  Value=contact_start_config
  Leg Gait FSM : Stateflow chart  TreatAsAtomicUnit=on
  "Velocity Transform Body -> Leg Origin" : Subsystem  mask{distance=distance, rotation_z=rotation_z}
      mask prompts: rotation_z "Rotation Z"
  config_cmd : Outport
  config_dot_cmd : Outport  Port=2
  velocity_control : Outport  Port=3
  wires:
  Leg Gait FSM/3(velocity_control) -> velocity_control/1
  Leg Gait FSM/1(config_cmd) -> config_cmd/1
  Leg Gait FSM/2(config_dot_cmd) -> config_dot_cmd/1
  "Velocity Transform Body -> Leg Origin"/1(vx_leg) -> Leg Gait FSM/1(vx)
  "Velocity Transform Body -> Leg Origin"/2(vy_leg) -> Leg Gait FSM/2(vy)
  "Velocity Transform Body -> Leg Origin"/3(omega) -> Leg Gait FSM/3(omega)
  normalised_time/1 -> Leg Gait FSM/4(u)
  vx_body/1 -> "Velocity Transform Body -> Leg Origin"/1(vx_body)
  vy_body/1 -> "Velocity Transform Body -> Leg Origin"/2(vy_body)
  omega_body/1 -> "Velocity Transform Body -> Leg Origin"/3(omega_body)
  leg_config/1 -> Leg Gait FSM/5(config)
  Constant/1 -> Leg Gait FSM/8(contact_start_config)
  phi/1 -> Leg Gait FSM/6(phi)
  beta/1 -> Leg Gait FSM/7(beta)

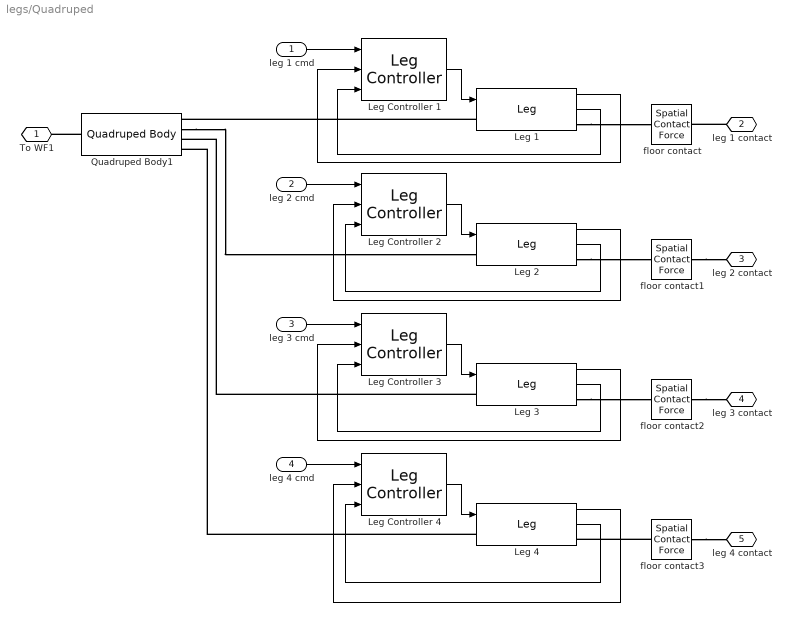
== system legs/Quadruped ==
  leg 1 cmd : Inport
  leg 2 cmd : Inport  Port=2
  leg 3 cmd : Inport  Port=3
  leg 4 cmd : Inport  Port=4
  Leg {1..4} (4 alike) : $bdroot/Leg  length_1=0.1  length_2=0.3  length_3=0.3  radius=0.02  mass_1=0.1  mass_2=0.3  mass_3=0.3
  Leg Controller {1..4} (4 alike) : $bdroot/Leg Controller  kp=[20; 20; 20]  ki=[5; 5; 5]  kd=[1; 1; 1]
  Quadruped Body1 : $bdroot/Quadruped Body  length=0.8  width=0.6  height=0.1  leg_radius=0.02  mass=0
      link override Rigid Transform: RotationAngle=90
  floor contact{,1..3} (4 alike) : sm_lib/Forces and Torques/Spatial Contact Force  CoefficientOfDynamicFriction=0.3  CoefficientOfStaticFriction=1  NormalDamping=1e3  NormalDampingUnits=N/(m/s)  NormalStiffness=1e6  NormalStiffnessUnits=N/m  FrictionalCriticalVelocity=1e-3  FrictionalCriticalVelocityUnits=m/s  ZeroCrossDetectContactStartAndEnd=off  SenseFrictionalForceMagnitude=off  SenseNormalForceMagnitude=off  SenseSeparationDistance=off  NormalTransitionRegionWidth=1e-4  NormalTransitionRegionWidthUnits=m  FrictionType=SmoothStickSlip
  To WF1 : PMIOPort  Side=Left
  leg 1 contact : PMIOPort  Port=2  Side=Right
  leg 2 contact : PMIOPort  Port=3  Side=Right
  leg 3 contact : PMIOPort  Port=4  Side=Right
  leg 4 contact : PMIOPort  Port=5  Side=Right
  wires:
  Leg Controller 2/1 -> Leg 2/1
  Leg Controller 3/1 -> Leg 3/1
  Leg 1/2 -> Leg Controller 1/3
  Leg Controller 1/1 -> Leg 1/1
  Leg 3/1 -> Leg Controller 3/2
  Leg 4/2 -> Leg Controller 4/3
  Leg Controller 4/1 -> Leg 4/1
  Leg 4/1 -> Leg Controller 4/2
  leg 3 cmd/1 -> Leg Controller 3/1
  leg 1 cmd/1 -> Leg Controller 1/1
  leg 4 cmd/1 -> Leg Controller 4/1
  Leg 3/2 -> Leg Controller 3/3
  leg 2 cmd/1 -> Leg Controller 2/1
  Leg 1/1 -> Leg Controller 1/2
  Leg 2/1 -> Leg Controller 2/2
  Leg 2/2 -> Leg Controller 2/3
  connections:
  Quadruped Body1/LConn1 -- To WF1/RConn1
  Leg 3/RConn1 -- floor contact2/LConn1
  floor contact3/LConn1 -- Leg 4/RConn1
  Leg 2/RConn1 -- floor contact1/LConn1
  Leg 4/LConn1 -- Quadruped Body1/RConn4
  Leg 1/LConn1 -- Quadruped Body1/RConn1
  Quadruped Body1/RConn2 -- Leg 2/LConn1
  Leg 3/LConn1 -- Quadruped Body1/RConn3
  Leg 1/RConn1 -- floor contact/LConn1
  leg 1 contact/RConn1 -- floor contact/RConn1
  floor contact2/RConn1 -- leg 3 contact/RConn1
  floor contact3/RConn1 -- leg 4 contact/RConn1
  floor contact1/RConn1 -- leg 2 contact/RConn1

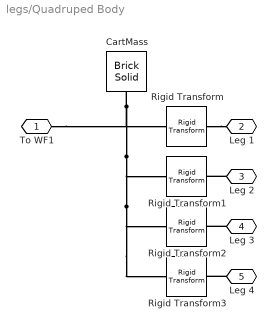
== system legs/Quadruped Body ==
  CartMass : sm_lib/Body Elements/Brick Solid  GraphicAmbientColor=[0.15 0.15 0.15 1.0]  BasedOnType=Mass  BrickDimensions=[length width height]  BrickDimensionUnits=m  CenterOfMass=[0 0 0]  CenterOfMassUnits=m  GraphicDiffuseColor=[0.8 0.0 0.2]  Density=1000  DensityUnits=kg/m^3  DoExposeReferenceFrame=on  GraphicEmissiveColor=[0.0 0.0 0.0 1.0]  ExportEntireGeometry=off  SerializedFrames=<Frames/>  MarkerShape=Sphere  MarkerSize=10  GraphicType=FromGeometry  InertiaType=CalculateFromGeometry  Mass=mass  MassUnits=kg  MomentsOfInertia=[1 1 1]  MomentsOfInertiaUnits=kg*m^2  GraphicOpacity=1.0  ProductsOfInertia=[0 0 0]  ProductsOfInertiaUnits=kg*m^2  GraphicShininess=75  GraphicSpecularColor=[0.5 0.5 0.5 1.0]  GraphicVisPropType=SimpleVisualProperties
  Rigid Transform : sm_lib/Frames and Transforms/Rigid Transform  TranslationMethod=Cartesian  TranslationStandardOffset=0  TranslationLengthUnit=m  TranslationStandardAxis=+Z  TranslationCartesianOffset=[length/2-leg_radius width/2 0]  TranslationROffset=0  TranslationROffsetUnits=m  TranslationZOffset=0  TranslationZOffsetUnits=m  TranslationThetaOffset=0  TranslationThetaOffsetUnits=deg  RotationMethod=StandardAxis  RotationAngleUnits=deg  RotationStandardAxis=+Z  RotationAngle=90  RotationArbitraryAxis=[0 0 1]  FollAlignAxisA=+X  BaseAlignAxisA=+Y  FollAlignAxisB=+Y  BaseAlignAxisB=+Z  RotationSequenceAxes=FollowerAxes  RotationSequence=XYX  RotationSequenceAngles=[0 0 0]  RotationSequenceAnglesUnits=deg  RotationMatrix=[1 0 0; 0 1 0; 0 0 1]
  Rigid Transform1 : sm_lib/Frames and Transforms/Rigid Transform  TranslationMethod=Cartesian  TranslationStandardOffset=0  TranslationLengthUnit=m  TranslationStandardAxis=+Z  TranslationCartesianOffset=[length/2-leg_radius -width/2 0]  TranslationROffset=0  TranslationROffsetUnits=m  TranslationZOffset=0  TranslationZOffsetUnits=m  TranslationThetaOffset=0  TranslationThetaOffsetUnits=deg  RotationMethod=StandardAxis  RotationAngleUnits=deg  RotationStandardAxis=+Z  RotationAngle=-90  RotationArbitraryAxis=[0 0 1]  FollAlignAxisA=+X  BaseAlignAxisA=+Y  FollAlignAxisB=+Y  BaseAlignAxisB=+Z  RotationSequenceAxes=FollowerAxes  RotationSequence=XYX  RotationSequenceAngles=[0 0 0]  RotationSequenceAnglesUnits=deg  RotationMatrix=[1 0 0; 0 1 0; 0 0 1]
  Rigid Transform2 : sm_lib/Frames and Transforms/Rigid Transform  TranslationMethod=Cartesian  TranslationStandardOffset=0  TranslationLengthUnit=m  TranslationStandardAxis=+Z  TranslationCartesianOffset=[-length/2+leg_radius width/2 0]  TranslationROffset=0  TranslationROffsetUnits=m  TranslationZOffset=0  TranslationZOffsetUnits=m  TranslationThetaOffset=0  TranslationThetaOffsetUnits=deg  RotationMethod=StandardAxis  RotationAngleUnits=deg  RotationStandardAxis=+Z  RotationAngle=90  RotationArbitraryAxis=[0 0 1]  FollAlignAxisA=+X  BaseAlignAxisA=+Y  FollAlignAxisB=+Y  BaseAlignAxisB=+Z  RotationSequenceAxes=FollowerAxes  RotationSequence=XYX  RotationSequenceAngles=[0 0 0]  RotationSequenceAnglesUnits=deg  RotationMatrix=[1 0 0; 0 1 0; 0 0 1]
  Rigid Transform3 : sm_lib/Frames and Transforms/Rigid Transform  TranslationMethod=Cartesian  TranslationStandardOffset=0  TranslationLengthUnit=m  TranslationStandardAxis=+Z  TranslationCartesianOffset=[-length/2+leg_radius -width/2 0]  TranslationROffset=0  TranslationROffsetUnits=m  TranslationZOffset=0  TranslationZOffsetUnits=m  TranslationThetaOffset=0  TranslationThetaOffsetUnits=deg  RotationMethod=StandardAxis  RotationAngleUnits=deg  RotationStandardAxis=+Z  RotationAngle=-90  RotationArbitraryAxis=[0 0 1]  FollAlignAxisA=+X  BaseAlignAxisA=+Y  FollAlignAxisB=+Y  BaseAlignAxisB=+Z  RotationSequenceAxes=FollowerAxes  RotationSequence=XYX  RotationSequenceAngles=[0 0 0]  RotationSequenceAnglesUnits=deg  RotationMatrix=[1 0 0; 0 1 0; 0 0 1]
  To WF1 : PMIOPort  Side=Left
  Leg 1 : PMIOPort  Port=2  Side=Right
  Leg 2 : PMIOPort  Port=3  Side=Right
  Leg 3 : PMIOPort  Port=4  Side=Right
  Leg 4 : PMIOPort  Port=5  Side=Right
  connections:
  Rigid Transform/RConn1 -- Leg 1/RConn1
  CartMass/RConn1 -- Rigid Transform1/LConn1 -- Rigid Transform3/LConn1 -- Rigid Transform2/LConn1 -- To WF1/RConn1 -- Rigid Transform/LConn1
  Leg 2/RConn1 -- Rigid Transform1/RConn1
  Leg 4/RConn1 -- Rigid Transform3/RConn1
  Leg 3/RConn1 -- Rigid Transform2/RConn1

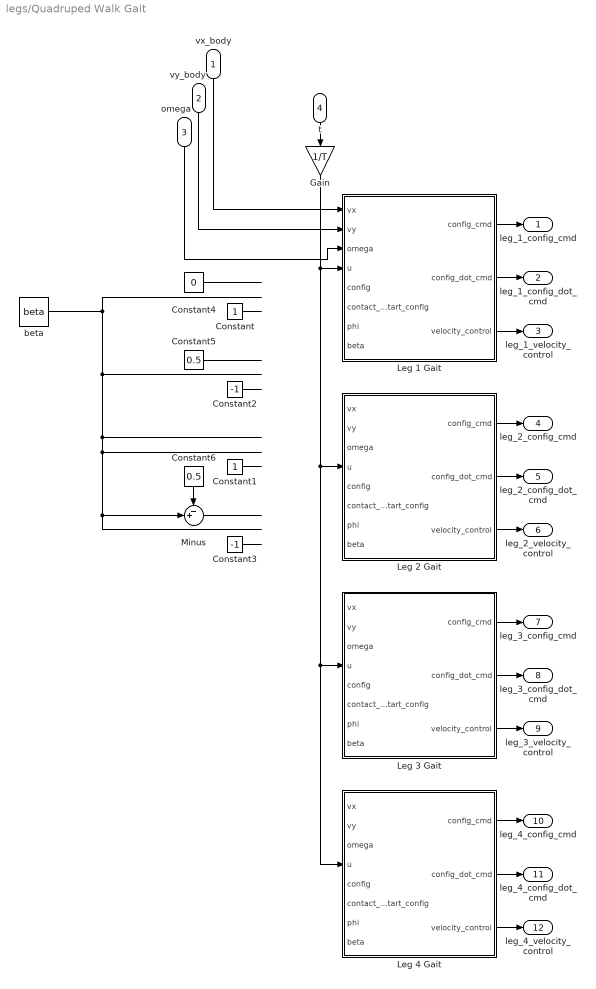
== system legs/Quadruped Walk Gait ==
  vx_body : Inport
  vy_body : Inport  Port=2
  omega : Inport  Port=3
  t : Inport  Port=4
  Constant : Constant
  Constant1 : Constant
  Constant2 : Constant  Value=-1
  Constant3 : Constant  Value=-1
  Constant4 : Constant  Value=0
  Constant5 : Constant  Value=0.5
  Constant6 : Constant  Value=0.5
  Gain : Gain  Gain=1/T
  Leg 1 Gait : Stateflow chart  TreatAsAtomicUnit=on
  Leg 2 Gait : Stateflow chart  TreatAsAtomicUnit=on
  Leg 3 Gait : Stateflow chart  TreatAsAtomicUnit=on
  Leg 4 Gait : Stateflow chart  TreatAsAtomicUnit=on
  Minus : Sum  Inputs=-+|
  beta : Constant  Value=beta
  leg_1_config_cmd : Outport
  leg_1_config_dot_cmd : Outport  Port=2
  leg_1_velocity_control : Outport  Port=3
  leg_2_config_cmd : Outport  Port=4
  leg_2_config_dot_cmd : Outport  Port=5
  leg_2_velocity_control : Outport  Port=6
  leg_3_config_cmd : Outport  Port=7
  leg_3_config_dot_cmd : Outport  Port=8
  leg_3_velocity_control : Outport  Port=9
  leg_4_config_cmd : Outport  Port=10
  leg_4_config_dot_cmd : Outport  Port=11
  leg_4_velocity_control : Outport  Port=12
  wires:
  Constant3/1 -> ?
  Leg 1 Gait/3(velocity_control) -> leg_1_velocity_control/1
  Constant5/1 -> ?
  Constant4/1 -> ?
  Constant1/1 -> ?
  Leg 1 Gait/2(config_dot_cmd) -> leg_1_config_dot_cmd/1
  t/1 -> Gain/1
  Minus/1 -> ?
  Constant2/1 -> ?
  beta/1 -> Minus/2
  Constant6/1 -> Minus/1
  Constant/1 -> ?
  Leg 1 Gait/1(config_cmd) -> leg_1_config_cmd/1
  vx_body/1 -> Leg 1 Gait/1(vx)
  vy_body/1 -> Leg 1 Gait/2(vy)
  omega/1 -> Leg 1 Gait/3(omega)
  Gain/1 -> Leg 4 Gait/4(u), Leg 3 Gait/4(u), Leg 2 Gait/4(u), Leg 1 Gait/4(u)
  Leg 2 Gait/1(config_cmd) -> leg_2_config_cmd/1
  Leg 2 Gait/2(config_dot_cmd) -> leg_2_config_dot_cmd/1
  Leg 2 Gait/3(velocity_control) -> leg_2_velocity_control/1
  Leg 3 Gait/1(config_cmd) -> leg_3_config_cmd/1
  Leg 3 Gait/2(config_dot_cmd) -> leg_3_config_dot_cmd/1
  Leg 3 Gait/3(velocity_control) -> leg_3_velocity_control/1
  Leg 4 Gait/1(config_cmd) -> leg_4_config_cmd/1
  Leg 4 Gait/2(config_dot_cmd) -> leg_4_config_dot_cmd/1
  Leg 4 Gait/3(velocity_control) -> leg_4_velocity_control/1

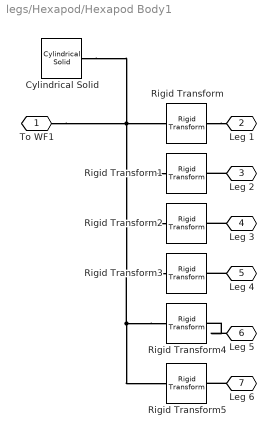
== system legs/Hexapod/Hexapod Body1 ==
  Cylindrical Solid : sm_lib/Body Elements/Cylindrical Solid  GraphicAmbientColor=[0.15 0.15 0.15 1.0]  BasedOnType=Density  CenterOfMass=[0 0 0]  CenterOfMassUnits=m  GraphicDiffuseColor=[0.5 0.5 0.5]  CylinderLength=height  CylinderLengthUnits=m  CylinderRadius=radius  CylinderRadiusUnits=m  Density=1000  DensityUnits=kg/m^3  DoExposeReferenceFrame=on  GraphicEmissiveColor=[0.0 0.0 0.0 1.0]  ExportEntireGeometry=off  SerializedFrames=<Frames/>  MarkerShape=Sphere  MarkerSize=10  GraphicType=FromGeometry  InertiaType=CalculateFromGeometry  Mass=1  MassUnits=kg  MomentsOfInertia=[1 1 1]  MomentsOfInertiaUnits=kg*m^2  GraphicOpacity=1.0  ProductsOfInertia=[0 0 0]  ProductsOfInertiaUnits=kg*m^2  GraphicShininess=75  GraphicSpecularColor=[0.5 0.5 0.5 1.0]  GraphicVisPropType=SimpleVisualProperties
  Rigid Transform : sm_lib/Frames and Transforms/Rigid Transform  TranslationMethod=Cylindrical  TranslationStandardOffset=0  TranslationLengthUnit=m  TranslationStandardAxis=+Z  TranslationCartesianOffset=[radius*cos(1/3*pi) radius*sin(1/3*pi) 0]  TranslationROffset=radius  TranslationROffsetUnits=m  TranslationZOffset=0  TranslationZOffsetUnits=m  TranslationThetaOffset=60  TranslationThetaOffsetUnits=deg  RotationMethod=StandardAxis  RotationAngleUnits=deg  RotationStandardAxis=+Z  RotationAngle=60  RotationArbitraryAxis=[0 0 1]  FollAlignAxisA=+X  BaseAlignAxisA=+Y  FollAlignAxisB=+Y  BaseAlignAxisB=+Z  RotationSequenceAxes=FollowerAxes  RotationSequence=XYX  RotationSequenceAngles=[0 0 0]  RotationSequenceAnglesUnits=deg  RotationMatrix=[1 0 0; 0 1 0; 0 0 1]
  Rigid Transform1 : sm_lib/Frames and Transforms/Rigid Transform  TranslationMethod=Cartesian  TranslationStandardOffset=0  TranslationLengthUnit=m  TranslationStandardAxis=+Z  TranslationCartesianOffset=[radius*cos(2/3*pi) radius*sin(2/3*pi) 0]  TranslationROffset=0  TranslationROffsetUnits=m  TranslationZOffset=0  TranslationZOffsetUnits=m  TranslationThetaOffset=0  TranslationThetaOffsetUnits=deg  RotationMethod=StandardAxis  RotationAngleUnits=rad  RotationStandardAxis=+Z  RotationAngle=2/3*pi  RotationArbitraryAxis=[0 0 1]  FollAlignAxisA=+X  BaseAlignAxisA=+Y  FollAlignAxisB=+Y  BaseAlignAxisB=+Z  RotationSequenceAxes=FollowerAxes  RotationSequence=XYX  RotationSequenceAngles=[0 0 0]  RotationSequenceAnglesUnits=deg  RotationMatrix=[1 0 0; 0 1 0; 0 0 1]
  Rigid Transform2 : sm_lib/Frames and Transforms/Rigid Transform  TranslationMethod=Cartesian  TranslationStandardOffset=0  TranslationLengthUnit=m  TranslationStandardAxis=+Z  TranslationCartesianOffset=[radius*cos(pi) radius*sin(pi) 0]  TranslationROffset=0  TranslationROffsetUnits=m  TranslationZOffset=0  TranslationZOffsetUnits=m  TranslationThetaOffset=0  TranslationThetaOffsetUnits=deg  RotationMethod=StandardAxis  RotationAngleUnits=rad  RotationStandardAxis=+Z  RotationAngle=pi  RotationArbitraryAxis=[0 0 1]  FollAlignAxisA=+X  BaseAlignAxisA=+Y  FollAlignAxisB=+Y  BaseAlignAxisB=+Z  RotationSequenceAxes=FollowerAxes  RotationSequence=XYX  RotationSequenceAngles=[0 0 0]  RotationSequenceAnglesUnits=deg  RotationMatrix=[1 0 0; 0 1 0; 0 0 1]
  Rigid Transform3 : sm_lib/Frames and Transforms/Rigid Transform  TranslationMethod=Cartesian  TranslationStandardOffset=0  TranslationLengthUnit=m  TranslationStandardAxis=+Z  TranslationCartesianOffset=[radius*cos(4/3*pi) radius*sin(4/3*pi) 0]  TranslationROffset=0  TranslationROffsetUnits=m  TranslationZOffset=0  TranslationZOffsetUnits=m  TranslationThetaOffset=0  TranslationThetaOffsetUnits=deg  RotationMethod=StandardAxis  RotationAngleUnits=rad  RotationStandardAxis=+Z  RotationAngle=4/3*pi  RotationArbitraryAxis=[0 0 1]  FollAlignAxisA=+X  BaseAlignAxisA=+Y  FollAlignAxisB=+Y  BaseAlignAxisB=+Z  RotationSequenceAxes=FollowerAxes  RotationSequence=XYX  RotationSequenceAngles=[0 0 0]  RotationSequenceAnglesUnits=deg  RotationMatrix=[1 0 0; 0 1 0; 0 0 1]
  Rigid Transform4 : sm_lib/Frames and Transforms/Rigid Transform  TranslationMethod=Cartesian  TranslationStandardOffset=0  TranslationLengthUnit=m  TranslationStandardAxis=+Z  TranslationCartesianOffset=[radius*cos(5/3*pi) radius*sin(5/3*pi) 0]  TranslationROffset=0  TranslationROffsetUnits=m  TranslationZOffset=0  TranslationZOffsetUnits=m  TranslationThetaOffset=0  TranslationThetaOffsetUnits=deg  RotationMethod=StandardAxis  RotationAngleUnits=rad  RotationStandardAxis=+Z  RotationAngle=5/3*pi  RotationArbitraryAxis=[0 0 1]  FollAlignAxisA=+X  BaseAlignAxisA=+Y  FollAlignAxisB=+Y  BaseAlignAxisB=+Z  RotationSequenceAxes=FollowerAxes  RotationSequence=XYX  RotationSequenceAngles=[0 0 0]  RotationSequenceAnglesUnits=deg  RotationMatrix=[1 0 0; 0 1 0; 0 0 1]
  Rigid Transform5 : sm_lib/Frames and Transforms/Rigid Transform  TranslationMethod=Cartesian  TranslationStandardOffset=0  TranslationLengthUnit=m  TranslationStandardAxis=+Z  TranslationCartesianOffset=[radius*cos(2*pi) radius*sin(2*pi) 0]  TranslationROffset=0  TranslationROffsetUnits=m  TranslationZOffset=0  TranslationZOffsetUnits=m  TranslationThetaOffset=0  TranslationThetaOffsetUnits=deg  RotationMethod=StandardAxis  RotationAngleUnits=rad  RotationStandardAxis=+Z  RotationAngle=2*pi  RotationArbitraryAxis=[0 0 1]  FollAlignAxisA=+X  BaseAlignAxisA=+Y  FollAlignAxisB=+Y  BaseAlignAxisB=+Z  RotationSequenceAxes=FollowerAxes  RotationSequence=XYX  RotationSequenceAngles=[0 0 0]  RotationSequenceAnglesUnits=deg  RotationMatrix=[1 0 0; 0 1 0; 0 0 1]
  To WF1 : PMIOPort  Side=Left
  Leg 1 : PMIOPort  Port=2  Side=Right
  Leg 2 : PMIOPort  Port=3  Side=Right
  Leg 3 : PMIOPort  Port=4  Side=Right
  Leg 4 : PMIOPort  Port=5  Side=Right
  Leg 5 : PMIOPort  Port=6  Side=Right
  Leg 6 : PMIOPort  Port=7  Side=Right
  connections:
  Rigid Transform/RConn1 -- Leg 1/RConn1
  Rigid Transform4/LConn1 -- Rigid Transform5/LConn1 -- To WF1/RConn1 -- Cylindrical Solid/RConn1 -- Rigid Transform/LConn1 -- Rigid Transform1/LConn1 -- Rigid Transform2/LConn1 -- Rigid Transform3/LConn1
  Leg 2/RConn1 -- Rigid Transform1/RConn1
  Leg 4/RConn1 -- Rigid Transform3/RConn1
  Leg 3/RConn1 -- Rigid Transform2/RConn1
  Leg 5/RConn1 -- Rigid Transform4/RConn1
  Leg 6/RConn1 -- Rigid Transform5/RConn1

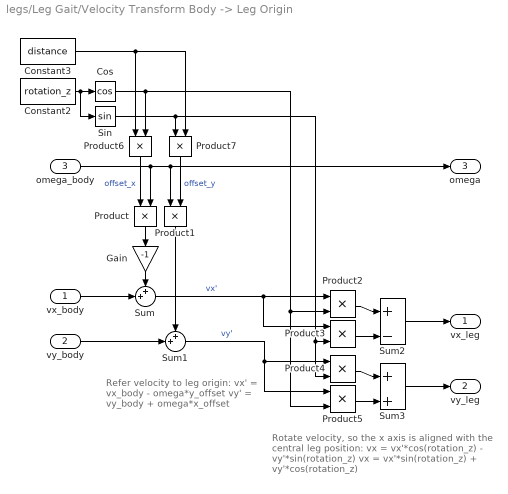
== system legs/Leg Gait/Velocity Transform Body -> Leg Origin ==
  note: Refer velocity to leg origin:
      | vx' = vx_body - omega*y_offset
      | vy' = vy_body + omega*x_offset
  note: Rotate velocity, so the x axis is aligned with the
      | central leg position:
      | vx = vx'*cos(rotation_z) - vy'*sin(rotation_z)
      | vx = vx'*sin(rotation_z) + vy'*cos(rotation_z)
  vx_body : Inport
  vy_body : Inport  Port=2
  omega_body : Inport  Port=3
  Constant2 : Constant  Value=rotation_z
  Constant3 : Constant  Value=distance
  Cos : Trigonometry  Operator=cos
  Gain : Gain  Gain=-1
  Product{,1..7} (8 alike) : Product
  Sin : Trigonometry
  Sum : Sum  Inputs=++|
  Sum1 : Sum  Inputs=++|
  Sum2 : Sum  Inputs=+|-
  Sum3 : Sum  Inputs=+|+
  vx_leg : Outport
  vy_leg : Outport  Port=2
  omega : Outport  Port=3
  wires:
  vx_body/1 -> Sum/2
  vy_body/1 -> Sum1/2
  Product/1 -> Gain/1
  Product1/1 -> Sum1/1
  Gain/1 -> Sum/1
  omega_body/1 -> Product/2, Product1/1, omega/1
  Product6/1 -> Product/1  "offset_x"
  Product7/1 -> Product1/2  "offset_y"
  Sum/1 -> Product3/1, Product2/1  "vx'"
  Sum1/1 -> Product5/1, Product4/1  "vy'"
  Constant2/1 -> Cos/1, Sin/1
  Product2/1 -> Sum2/1
  Product3/1 -> Sum2/2
  Product5/1 -> Sum3/2
  Product4/1 -> Sum3/1
  Cos/1 -> Product5/2, Product2/2, Product6/2
  Sin/1 -> Product4/2, Product3/2, Product7/1
  Sum2/1 -> vx_leg/1
  Sum3/1 -> vy_leg/1
  Constant3/1 -> Product6/1, Product7/2

== stateflow chart legs/Quadruped Walk Gait/Leg 3 Gait ==
  state Initial_
    entry:
    u_start = u;
    u_elapsed = 0;
    during:
    u_elapsed = u - u_start;
  state Lifted
    entry:
    N = 10;
    waypoints = leg_waypoints(config, contact_start_config, N);
    u_start = u;
    u_elapsed = 0;
    velocity_control = 0;
    during:
    i = ceil((u_elapsed/(1-beta))*N);
    config_cmd = waypoints(i);
  state Contact
    entry:
    u_start = u;
    u_elapsed = 0;
    velocity_control = 1;
    during:
    config_dot_cmd = leg_config_dot_ik(config, vx, vy, omega);
    u_elapsed = u - u_start;
  (default) -> Initial_
  Initial_ -> Contact : [u_elapsed > phi]
  Contact -> Lifted : [u_elapsed > beta]
  Lifted -> Contact : [u_elapsed > (1-beta)]
  data: config_cmd output; config_dot_cmd output; vx input; vy input; omega input; u input; velocity_control output; N local; config input; i local; u_elapsed local; u_start local; waypoints local; contact_start_config input; phi input; beta input

== stateflow chart legs/Quadruped Walk Gait/Leg 4 Gait ==
  state Initial_
    entry:
    u_start = u;
    u_elapsed = 0;
    during:
    u_elapsed = u - u_start;
  state Lifted
    entry:
    N = 10;
    waypoints = leg_waypoints(config, contact_start_config, N);
    u_start = u;
    u_elapsed = 0;
    velocity_control = 0;
    during:
    i = ceil((u_elapsed/(1-beta))*N);
    config_cmd = waypoints(i);
  state Contact
    entry:
    u_start = u;
    u_elapsed = 0;
    velocity_control = 1;
    during:
    config_dot_cmd = leg_config_dot_ik(config, vx, vy, omega);
    u_elapsed = u - u_start;
  (default) -> Initial_
  Initial_ -> Contact : [u_elapsed > phi]
  Contact -> Lifted : [u_elapsed > beta]
  Lifted -> Contact : [u_elapsed > (1-beta)]
  data: config_cmd output; config_dot_cmd output; vx input; vy input; omega input; u input; velocity_control output; N local; config input; i local; u_elapsed local; u_start local; waypoints local; contact_start_config input; phi input; beta input

== stateflow chart legs/Leg Gait/Leg Gait FSM ==
  state Initial_
    entry:
    u_start = u;
    u_elapsed = 0;
    during:
    u_elapsed = u - u_start;
  state Lifted
    entry:
    N = 10;
    waypoints = leg_waypoints(config, contact_start_config, N);
    u_start = u;
    u_elapsed = 0;
    velocity_control = 0;
    during:
    i = ceil((u_elapsed/(1-beta))*N);
    config_cmd = waypoints(i);
  state Contact
    entry:
    u_start = u;
    u_elapsed = 0;
    velocity_control = 1;
    during:
    config_dot_cmd = leg_config_dot_ik(config, vx, vy, omega);
    u_elapsed = u - u_start;
  (default) -> Initial_
  Initial_ -> Contact : [u_elapsed > phi]
  Contact -> Lifted : [u_elapsed > beta]
  Lifted -> Contact : [u_elapsed > (1-beta)]
  data: config_cmd output; config_dot_cmd output; vx input; vy input; omega input; u input; velocity_control output; N local; config input; i local; u_elapsed local; u_start local; waypoints local; phi input; beta input; contact_start_config input

== stateflow chart legs/Quadruped Walk Gait/Leg 1 Gait ==
  state Initial_
    entry:
    u_start = u;
    u_elapsed = 0;
    during:
    u_elapsed = u - u_start;
  state Lifted
    entry:
    N = 10;
    waypoints = leg_waypoints(config, contact_start_config, N);
    u_start = u;
    u_elapsed = 0;
    velocity_control = 0;
    during:
    i = ceil((u_elapsed/(1-beta))*N);
    config_cmd = waypoints(i);
  state Contact
    entry:
    u_start = u;
    u_elapsed = 0;
    velocity_control = 1;
    during:
    config_dot_cmd = leg_config_dot_ik(config, vx, vy, omega);
    u_elapsed = u - u_start;
  (default) -> Initial_
  Initial_ -> Contact : [u_elapsed > phi]
  Contact -> Lifted : [u_elapsed > beta]
  Lifted -> Contact : [u_elapsed > (1-beta)]
  data: config_cmd output; config_dot_cmd output; vx input; vy input; omega input; u input; velocity_control output; N local; config input; i local; u_elapsed local; u_start local; waypoints local; contact_start_config input; phi input; beta input
